simulink model "ASG_algorithm"  (R2024a)
settings: Solver=ode1  StartTime=0.0  StopTime=60  FixedStep=0.01  RelTol=1e-3
libraries: simulink x3
(part 1 of 3)
settings Model: Creator=victo  LastModifiedBy=victo

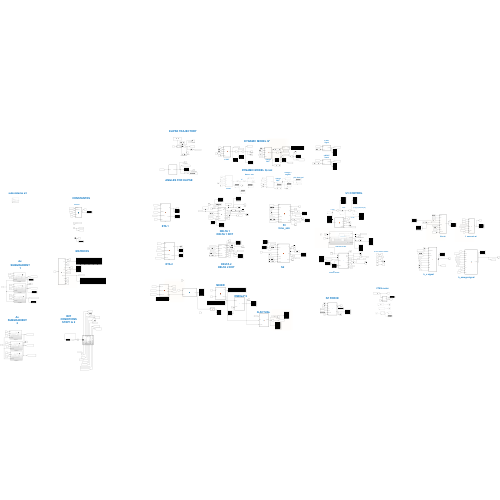
[thumbnail: Simulink's stored preview of the top-level diagram]
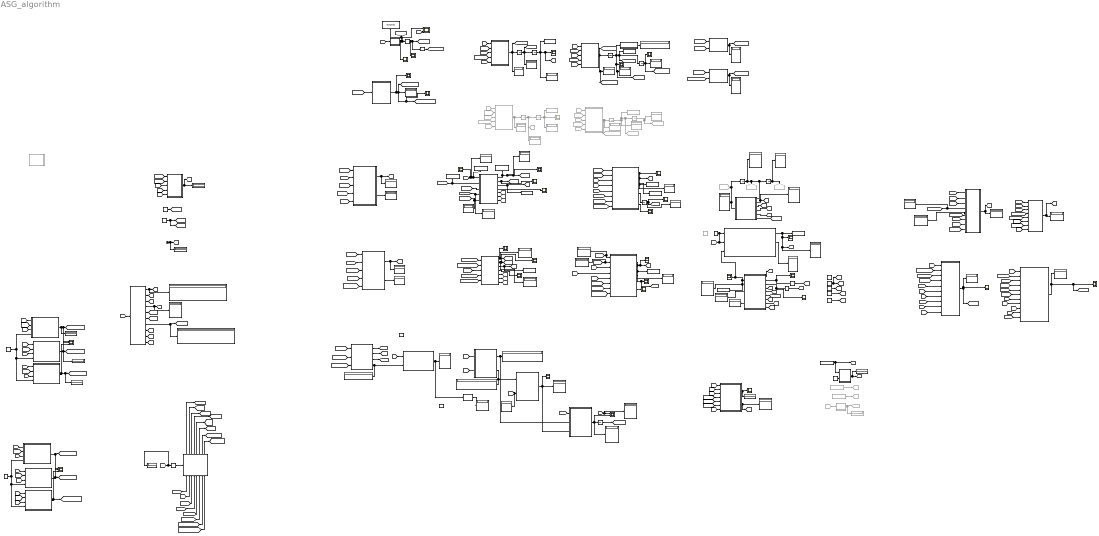
== system ASG_algorithm ==
  note: omega DOT
  note: q_dot
  note: h_omega signal
  note: ETA 2
  note: DYNAMIC MODEL Q*
  note: S1
  note: DELTA 1
      | DELTA 1 DOT
  note: h_v signal
  note: U1 CONTROL
  note: S2
  note: U1
      | CONTROL SIGNAL
  note: MATRICES
  note: Av. SUBGRADIENT 2
  note: S1
      | time_sim
  note: Av. SUBGRADIENT 1
  note: Q = Q*
  note: ELIPSE TRAJECTORY
  note: LOW PASS FILTER
  note: DELTA 2
      | DELTA 2 DOT
  note: fv(v,w)
  note: CONSTANTES
  note: V DOT
  note: f_omega(v,w)
  note: RHO & K1
  note: ETA 1
  note: K1, K2, THETA1, THETA2
  note: ANGLES FOR ELIPSE
  note: INIT CONDITIONS
      | STEP1 & 2
  note: DYNAMIC MODEL Q real
  note: V DOT
  note: omega DOT
  note: S1
  note: Kappa - pos
  note: omega, v angular
  note: phi, theta, psi
  note: q = [x,y,z,phi,theta,psi]
  note: V
  note: q_ddot
  note: MIXER
  note: CTES motor
  note: OMEGA^2
  note: subsistema s3
  note: Q ACTUAL
  note: FZ FORCE
  note: q DOT signal
  note: q DDOT signal
  AverageBlock : Subsystem
  AverageBlock1 : Subsystem
  AverageBlock2 : Subsystem
  AverageBlock3 : Subsystem
  AverageBlock4 : Subsystem
  AverageBlock5 : Subsystem
  Clock : Clock
  Compare To Constant : simulink/Logic and Bit Operations/Compare To Constant  relop===  const=0.0  OutDataTypeStr=boolean
  Constant : Constant  Value=0.5
  Constant1 : Constant  Value=[0;0;0]
  Constant10 : Constant
  Constant14 : Constant  Commented=on  Value=2*10^(-4)
  Constant15 : Constant  Commented=on  Value=1.95*10^(-4)  VectorParams1D=off
  Constant16 : Constant  Value=5  VectorParams1D=off
  Constant2 : Constant  Value=[1;1;1;1]
  Constant3 : Constant  Value=[0;0;6;0;0;0]
  Constant4 : Constant  Value=4  VectorParams1D=off
  Constant5 : Constant  Value=0.03
  Constant7 : Constant  Value=6*10^(-4)
  Constant9 : Constant
  DELTA 1 : Scope
  DELTA 2 : Scope
  DELTA1_DOT : Scope
  DELTA2 DOT4 : Scope
  Derivative1 : Derivative
  Derivative2 : Derivative
  Display{,1..53,64..65,67..69,71,89} (61 alike) : Display
  Display{55,70,73..75,77..78} (7 alike) : Display  Commented=on
  Enabled Subsystem : Subsystem  TreatAsAtomicUnit=on
  From125 : From  Commented=on  GotoTag=FV
  From126 : From  Commented=on  GotoTag=ZERO_I
  From134 : From  Commented=on  GotoTag=I_ZERO
  From146 : From  Commented=on  GotoTag=D_INV
  From147 : From  Commented=on  GotoTag=Q_ACTUAL
  From148 : From  Commented=on  GotoTag=XIsubk
  From157 : From  Commented=on  GotoTag=FW
  From199 : From  Commented=on  GotoTag=JM
  From217 : From  Commented=on  GotoTag=D_INV
  From218 : From  Commented=on  GotoTag=Q_ACTUAL
  From219 : From  Commented=on  GotoTag=XIsubk
  Fz : Scope
  Goto103 : Goto  Commented=on  GotoTag=DM
  Goto104 : Goto  Commented=on  GotoTag=JM
  Goto105 : Goto  Commented=on  GotoTag=JM_INV
  Goto138 : Goto  Commented=on  GotoTag=ANGLES_Q_DOT
  Goto139 : Goto  Commented=on  GotoTag=ANGLES_Q_DDOT
  Goto140 : Goto  Commented=on  GotoTag=V_LIN
  Goto37 : Goto  Commented=on  GotoTag=q_signal
  Goto38 : Goto  Commented=on  GotoTag=q_dot_signal
  Goto47 : Goto  Commented=on  GotoTag=ANGLES_Q
  Goto63 : Goto  Commented=on  GotoTag=q_ddot_signal
  HV : Scope
  HW : Scope
  Integrator{,1..6} (7 alike) : Integrator
  Integrator{9..12} (4 alike) : Integrator  Commented=on
  KAPPA : Scope
  KAPPA POS DESEADA : Scope
  KAPPA REAL1 : Scope
  KAPPA REAL2 : Scope  Commented=on
  KAPPA des : Scope  NumInputPorts=2
  MATLAB Function : MATLAB Function  TreatAsAtomicUnit=on
  MATLAB Function1 : MATLAB Function  TreatAsAtomicUnit=on
  MATLAB Function10 : MATLAB Function  TreatAsAtomicUnit=on
  MATLAB Function11 : MATLAB Function  TreatAsAtomicUnit=on
  MATLAB Function12 : MATLAB Function  TreatAsAtomicUnit=on
  MATLAB Function13 : MATLAB Function  TreatAsAtomicUnit=on
  MATLAB Function14 : MATLAB Function  TreatAsAtomicUnit=on
  MATLAB Function15 : MATLAB Function  TreatAsAtomicUnit=on
  MATLAB Function16 : MATLAB Function  TreatAsAtomicUnit=on
  MATLAB Function17 : MATLAB Function  TreatAsAtomicUnit=on
  MATLAB Function18 : MATLAB Function  TreatAsAtomicUnit=on
  MATLAB Function19 : MATLAB Function  TreatAsAtomicUnit=on
  MATLAB Function2 : MATLAB Function  TreatAsAtomicUnit=on
  MATLAB Function20 : MATLAB Function  TreatAsAtomicUnit=on
  MATLAB Function21 : MATLAB Function  TreatAsAtomicUnit=on
  MATLAB Function22 : MATLAB Function  TreatAsAtomicUnit=on
  MATLAB Function23 : MATLAB Function  TreatAsAtomicUnit=on
  MATLAB Function24 : MATLAB Function  TreatAsAtomicUnit=on
  MATLAB Function25 : MATLAB Function  TreatAsAtomicUnit=on
  MATLAB Function26 : MATLAB Function  Commented=on  TreatAsAtomicUnit=on
  MATLAB Function27 : MATLAB Function  TreatAsAtomicUnit=on
  MATLAB Function28 : MATLAB Function  Commented=on  TreatAsAtomicUnit=on
  MATLAB Function3 : MATLAB Function  TreatAsAtomicUnit=on
  MATLAB Function4 : MATLAB Function  TreatAsAtomicUnit=on
  MATLAB Function45 : MATLAB Function  TreatAsAtomicUnit=on
  MATLAB Function5 : MATLAB Function  Commented=on  TreatAsAtomicUnit=on
  MATLAB Function6 : MATLAB Function  TreatAsAtomicUnit=on
  MATLAB Function7 : MATLAB Function  TreatAsAtomicUnit=on
  MATLAB Function8 : MATLAB Function  TreatAsAtomicUnit=on
  MATLAB Function9 : MATLAB Function  TreatAsAtomicUnit=on
  MIU1 : Constant  Value=0.02
  MIU2 : Constant  Commented=on  Value=0.1
  NORM D1 : Scope
  NORM S1 : Scope
  NORM S2 : Scope
  Norm D2 : Scope
  Q FILTRADA = Q ESTRELLA : Scope
  "Q SIGNAL " : Scope
  Q_comparing : Scope  NumInputPorts=2
  ROTORS VEL : Scope
  S1 : Scope
  S2 : Scope
  SIGN : Signum
  SIGN S1 : Scope
  SIGN S2 : Scope
  Scope1 : Scope  NumInputPorts=3
  Scope2 : Scope  NumInputPorts=3
  Scope3 : Scope
  Scope4 : Scope
  Sign1 : Signum
  Subsystem : Subsystem
  Subsystem1 : Subsystem  Commented=on
  THETA DESIRED : Scope
  THETA DOT DESIRED : Scope
  To Workspace : ToWorkspace  VariableName=dronepos  SampleTime=-1
  To Workspace1 : ToWorkspace  VariableName=simout1  SampleTime=-1
  To Workspace10 : ToWorkspace  VariableName=u1  SaveFormat=Timeseries  SampleTime=-1
  To Workspace11 : ToWorkspace  VariableName=kappad1  SampleTime=-1
  To Workspace13 : ToWorkspace  VariableName=q_star  SampleTime=-1
  To Workspace14 : ToWorkspace  Commented=on  VariableName=droneor1  SampleTime=-1
  To Workspace15 : ToWorkspace  Commented=on  VariableName=dronepos1  SampleTime=-1
  To Workspace2 : ToWorkspace  VariableName=s1  SampleTime=-1
  To Workspace3 : ToWorkspace  VariableName=time_sim  SampleTime=-1
  To Workspace4 : ToWorkspace  VariableName=kappad  SampleTime=-1
  To Workspace5 : ToWorkspace  VariableName=a1  SampleTime=-1
  To Workspace6 : ToWorkspace  VariableName=realkappa  SampleTime=-1
  To Workspace7 : ToWorkspace  VariableName=droneor  SampleTime=-1
  To Workspace8 : ToWorkspace  VariableName=a2  SampleTime=-1
  To Workspace9 : ToWorkspace  VariableName=s2  SampleTime=-1
  Unit Delay : UnitDelay  SampleTime=-1  HasFrameUpgradeWarning=on
  VEL DESEADA : Scope
  ZETA1 : Scope
  ZETA2 : Scope
  eta1 : MATLAB Function  TreatAsAtomicUnit=on
  eta2 : MATLAB Function  TreatAsAtomicUnit=on
  theta1 : Constant  Value=0.01
  theta2 : Constant  Value=0.5
  theta5 : Constant  Value=1e-6
  wires:
  MATLAB Function3/6(a1_y) -> [A1_Y]
  MATLAB Function11/1(fw) -> Display19/1, [FW]
  [TIME] -> MATLAB Function16/10(t)
  [KAPPA] -> Enabled Subsystem/2(kappa)
  [A1] -> MATLAB Function16/6(a1)
  MATLAB Function19/1(s2) -> Display42/1, To Workspace9/1, S2/1, [S2]
  [RHO1] -> MATLAB Function4/5(rho1)
  MATLAB Function6/2(t_s1) -> To Workspace3/1
  Enabled Subsystem/1(v_actual0) -> [V_ACT_0]
  [THETA2] -> MATLAB Function18/6(theta2)
  [V_ACTUAL] -> Display17/1, MATLAB Function10/4(v)
  [THETA2] -> AverageBlock3/2(theta)
  Enabled Subsystem/2(kappa0) -> [KAPPA_0]
  MATLAB Function6/3(Z1) -> Integrator2/1
  Integrator4/1 -> MATLAB Function7/1(vector_rpy), Integrator6/1, To Workspace7/1, [OMEGA_ACTV1], Scope3/1, [ANGLES_Q_DOT], Display21/1
  [THETA_ACTUAL] -> Enabled Subsystem/5(theta_actual)
  [G_Q] -> MATLAB Function10/6(g_q)
  [XIsubk] -> MATLAB Function14/5(xi_subv)
  From217/1 -> MATLAB Function28/3(D_inv)
  MATLAB Function17/1(omega_dot) -> [THETA_ACTUAL_DDOT], [ANGLES_Q_DDOT], Display25/1, Integrator4/1
  MATLAB Function8/6(a2_y) -> [A2_Y]
  MATLAB Function9/6(zero_I) -> [ZERO_I]
  [D_INV] -> MATLAB Function17/3(D_inv)
  From126/1 -> MATLAB Function28/2(zero_I)
  [A2X_AVERAGE] -> MATLAB Function19/6(a2x_average)
  From146/1 -> MATLAB Function5/3(D_inv)
  Integrator11/1 -> To Workspace15/1, KAPPA REAL2/1, Display78/1
  [K1] -> MATLAB Function12/4(k1)
  [THETA2] -> AverageBlock4/2(theta)
  From134/1 -> MATLAB Function5/2(I_zero)
  eta1/2(sum_result) -> Display9/1
  [TIME] -> AverageBlock1/3(t)
  Integrator6/1 -> Scope4/1, [THETA_ACTUAL], Display28/1
  [ETA1] -> MATLAB Function16/7(eta1)
  [S1] -> SIGN/1
  MATLAB Function/1(out) -> Display2/1, Integrator/1, Goto63/1
  AverageBlock5/1(Out1) -> [A2Z_AVERAGE], Scope2/3
  [ZETA1] -> MATLAB Function16/9(zeta1)
  [H_OMEGA] -> MATLAB Function12/6(h_omega)
  [OMEGA_ACTV1] -> MATLAB Function8/4(omega_actual)
  [DELTA1] -> MATLAB Function6/1(delta1)
  [RHO2] -> MATLAB Function12/7(k2)
  eta2/1(eta2) -> [ETA2], Display40/1
  [DELTA1] -> MATLAB Function16/8(delta1)
  [DELTA1_DOT] -> MATLAB Function6/2(delta1_dot)
  [TIME] -> AverageBlock5/3(t)
  [KAPPA] -> KAPPA/1, Display6/1, To Workspace6/1, MATLAB Function3/1(kappa_actual)
  MATLAB Function9/4(g_q) -> Display27/1, [G_Q]
  [A1Z_AVERAGE] -> MATLAB Function6/8(a1z_average)
  From147/1 -> MATLAB Function5/4(Q)
  [D_INV] -> MATLAB Function11/2(D_inv)
  MATLAB Function9/5(I_zero) -> [I_ZERO]
  MATLAB Function5/1(v_dot) -> Integrator9/1, Display73/1
  [S2] -> MATLAB Function12/9(s2)
  [V_ACTUAL] -> MATLAB Function11/4(v)
  [V_DESEADA] -> Display30/1, MATLAB Function3/5(v_desired)
  [TIME] -> MATLAB Function18/7(t)
  MATLAB Function3/5(a1_x) -> [A1_X]
  [C_q] -> MATLAB Function11/3(C)
  MATLAB Function3/2(delta1_dot) -> [DELTA1_DOT], DELTA1_DOT/1
  [S2] -> Sign1/1
  Integrator/1 -> Display4/1, Goto38/1, MATLAB Function/1(q_dot), Integrator1/1
  MATLAB Function8/5(a2_x) -> [A2_X]
  [I_ZERO] -> MATLAB Function14/2(I_zero)
  MATLAB Function8/4(F_d2) -> Norm D2/1
  [THETA2] -> eta2/1(theta2)
  [V_ACTUAL] -> Enabled Subsystem/1(v_actual)
  [A2_Y] -> AverageBlock4/1(In1)
  [FV] -> MATLAB Function16/1(fv)
  AverageBlock/1(Out1) -> Display33/1, [A1X_AVERAGE], Scope1/1
  MATLAB Function16/1(hv) -> [H_V], Display36/1, HV/1
  MATLAB Function3/4(F_d1) -> NORM D1/1
  [KFC0] -> MATLAB Function10/7(kf_c0)
  [KFC0] -> MATLAB Function11/8(Kf_c0)
  [A1_Y] -> AverageBlock1/1(In1)
  Enabled Subsystem/6(thetadot0) -> [THETADOT0]
  [ETA1] -> MATLAB Function6/3(eta1)
  theta2/1 -> [THETA2]
  MATLAB Function12/3(value_s2) -> Display71/1
  [OMEGA_ACTV1] -> MATLAB Function11/5(omega)
  [KAPPA_TRY] -> Enabled Subsystem/4(kappa_try)
  [TIME] -> MATLAB Function20/1(t)
  MATLAB Function21/1(desired_theta) -> THETA DESIRED/1, [DESIRED_THETA_ELIP], THETA DOT DESIRED/1, [DESIRED_DTHETA_ELIP], Display13/1
  Integrator12/1 -> Goto47/1, Display77/1
  Integrator2/1 -> Display/1, ZETA1/1, [ZETA1]
  [Q] -> MATLAB Function14/4(Q)
  [A2_Z] -> AverageBlock5/1(In1)
  [THETA0] -> eta2/2(THETA_0)
  [THETA_ACTUAL] -> MATLAB Function8/1(theta_actual)
  [S1] -> MATLAB Function12/8(s1)
  [THETA1] -> AverageBlock1/2(theta)
  AverageBlock2/1(Out1) -> Display1/1, [A1Z_AVERAGE], Scope1/3
  [TIME] -> MATLAB Function6/4(t)
  Constant1/1 -> [XIsubk], [XIsubk_dot]
  [DELTA2] -> MATLAB Function19/1(delta2), Display7/1
  From125/1 -> MATLAB Function5/1(fv)
  [D_INV] -> MATLAB Function14/3(D_inv)
  eta2/2(sum_result) -> Display41/1
  MATLAB Function12/1(u1) -> To Workspace10/1, Display43/1, "Q SIGNAL "/1, Subsystem/3(U1)
  [D] -> MATLAB Function12/1(D)
  Sign1/1 -> SIGN S2/1, MATLAB Function12/3(sign_s2)
  [DESIRED_DTHETA_ELIP] -> MATLAB Function8/5(omega_desired)
  [FW] -> MATLAB Function18/1(fw)
  [Q] -> MATLAB Function17/4(Q)
  MATLAB Function9/3(C) -> [C_q]
  Constant9/1 -> AverageBlock2/4(constant sign), AverageBlock1/4(constant sign), AverageBlock/4(constant sign)
  [D_INV] -> MATLAB Function10/2(D_inv)
  [A2Y_AVERAGE] -> MATLAB Function19/7(a2y_average)
  [DELTA2_DOT] -> Display65/1, MATLAB Function19/2(delta2_dot)
  Subsystem/1(Q_STAR) -> [Q], Display64/1, Q FILTRADA = Q ESTRELLA/1, To Workspace13/1
  [XIsubk] -> MATLAB Function17/5(xi_subw)
  theta1/1 -> [THETA1]
  Derivative2/1 -> [V_DOT_DESEADA]
  [ZERO_I] -> MATLAB Function17/2(zero_I)
  [EPSILON] -> MATLAB Function8/3(epsilon)
  [A2] -> MATLAB Function18/8(a2)
  [TIME] -> MATLAB Function19/4(t)
  [THETA_DES0] -> eta2/3(THETA_deseada_0)
  [TIME] -> AverageBlock4/3(t)
  AverageBlock4/1(Out1) -> [A2Y_AVERAGE], Scope2/2
  [THETA1] -> MATLAB Function4/4(theta1)
  [TIME] -> Compare To Constant/1, Display51/1
  [THETA1] -> MATLAB Function16/5(theta1)
  Compare To Constant/1 -> Enabled Subsystem/Enable
  [ZETA2] -> MATLAB Function18/5(zeta2)
  [DRAG_MATRIX] -> MATLAB Function/6(drag_matrix)
  [V_ACTUAL] -> MATLAB Function16/3(v_actual)
  [OMEGA_ACTV1] -> MATLAB Function18/2(omega)
  [THETA1] -> eta1/1(theta1)
  [OMEGA_ACTV1] -> Enabled Subsystem/6(omega_actual)
  [THETA1] -> MATLAB Function6/5(theta1)
  MATLAB Function7/1(R_graph) -> Display26/1
  [KAPPA_TRY] -> To Workspace4/1, MATLAB Function3/2(kappa_desired)
  [C_q] -> MATLAB Function/4(C_q)
  MIU1/1 -> [MIU], Subsystem/2(MIU2), Subsystem/1(MIU1)
  [THETADOT_DES0] -> eta2/5(THETA_DOT_0)
  theta5/1 -> [EPSILON]
  [DELTA2] -> MATLAB Function18/3(delta2)
  [TIME] -> AverageBlock2/3(t)
  [A1_Z] -> AverageBlock2/1(a1_z)
  [DRAG_MATRIX] -> MATLAB Function11/7(drag_matrix)
  [V_ACT_0] -> eta1/2(v_0)
  AverageBlock1/1(Out1) -> Scope1/2, Display29/1, [A1Y_AVERAGE]
  [KAPPA] -> KAPPA des/2
  [FW] -> MATLAB Function17/1(fw)
  Integrator10/1 -> To Workspace14/1, Goto138/1, Integrator12/1, Display74/1
  MATLAB Function19/2(Z2) -> [ZETA2], ZETA2/1
  MATLAB Function20/1(kappa) -> KAPPA des/1, Derivative1/1, To Workspace11/1, [KAPPA_TRY], KAPPA POS DESEADA/1
  Enabled Subsystem/8(thetadot_desired0) -> [THETADOT_DES0]
  MATLAB Function10/1(fv) -> [FV], Display23/1
  [OMEGA_ACTV1] -> Display18/1, MATLAB Function10/5(omega)
  MATLAB Function6/4(norm_s1) -> NORM S1/1
  Integrator1/1 -> Display3/1, Goto37/1
  SIGN/1 -> MATLAB Function12/2(sign_s1), SIGN S1/1
  [ZERO_I] -> MATLAB Function18/11(zero_I)
  [THETA2] -> MATLAB Function19/5(theta2)
  [TIME] -> MATLAB Function4/3(t)
  [A2Z_AVERAGE] -> MATLAB Function19/8(a2z_average)
  MATLAB Function9/8(l_arm) -> [L_ARM]
  [THETADOT0] -> eta2/4(THETA_DOT_desired_0)
  MATLAB Function9/7(drag_matrix) -> Display53/1, [DRAG_MATRIX]
  [D_INV] -> MATLAB Function18/9(D_inv)
  [XIsubk] -> MATLAB Function4/1(xi_subkappa)
  [A2_X] -> AverageBlock3/1(a2_x)
  MATLAB Function12/2(value_s1) -> Display68/1
  [DESIRED_THETA_ELIP] -> Enabled Subsystem/7(theta_desired)
  [KAPPA_0] -> eta1/5(kappa_0)
  Derivative1/1 -> VEL DESEADA/1, [V_DESEADA], Derivative2/1
  [TIME] -> AverageBlock3/3(t)
  [KA] -> MATLAB Function9/1("Ka ")
  [THETA1] -> AverageBlock2/2(theta)
  eta1/1(eta1) -> [ETA1], Display5/1
  [DESIRED_DTHETA_ELIP] -> Enabled Subsystem/8(thetadot_desired)
  [KAPPAD0] -> eta1/4(kappa_desired_0)
  [G_Q] -> MATLAB Function11/6(g_q)
  [XIsubk_dot] -> MATLAB Function4/2(xi_subkappa_dot)
  [TIME] -> AverageBlock/3(t)
  [V_DESEADA] -> MATLAB Function16/4(v_deseada)
  MATLAB Function8/2(delta2_dot) -> Display39/1, DELTA2 DOT4/1, [DELTA2_DOT]
  MATLAB Function9/1(D) -> Display24/1, [D]
  [A1_X] -> AverageBlock/1(a1_x)
  [EPSILON] -> MATLAB Function3/3(epsilon)
  [A1X_AVERAGE] -> MATLAB Function6/6(a1x_average)
  [C_q] -> MATLAB Function10/3(C)
  Enabled Subsystem/3(vdesired0) -> [V_DESIRED0]
  [G_Q] -> MATLAB Function/5(g_q)
  Constant10/1 -> AverageBlock3/4(constant sign), AverageBlock5/4(constant sign), AverageBlock4/4(constant sign)
  MATLAB Function6/1(s1) -> Display10/1, To Workspace2/1, [S1], S1/1
  [A1Y_AVERAGE] -> MATLAB Function6/7(a1y_average)
  [DESIRED_THETA_ELIP] -> MATLAB Function8/2(theta_desired)
  From219/1 -> MATLAB Function28/5(xi_subw)
  Integrator5/1 -> [KAPPA], KAPPA REAL1/1, Display31/1, To Workspace/1
  [H_V] -> MATLAB Function12/5(h_v)
  [Q] -> MATLAB Function18/10(Q)
  MATLAB Function14/1(v_dot) -> [V_DOT_ACTUAL], Display20/1, Integrator3/1
  Enabled Subsystem/5(theta0) -> [THETA0]
  Enabled Subsystem/7(theta_desired0) -> [THETA_DES0]
  [V_DESIRED0] -> eta1/3(v_deseada_0)
  [I_ZERO] -> MATLAB Function10/1(I_zero)
  MATLAB Function3/7(a1_z) -> [A1_Z]
  [ZERO_I] -> MATLAB Function11/1(zero_I)
  [V_ACTUAL] -> Display14/1, MATLAB Function3/4(v_actual)
  From148/1 -> MATLAB Function5/5(xi_subv)
  Enabled Subsystem/4(kappaD0) -> [KAPPAD0]
  [V_DESEADA] -> MATLAB Function21/1(des_vel)
  [V_DOT_DESEADA] -> MATLAB Function16/2(v_dot_deseada)
  [D_INV] -> MATLAB Function/3(D_inv)
  Constant/1 -> [KA]
  From218/1 -> MATLAB Function28/4(Q)
  [THETA2] -> AverageBlock5/2(theta)
  [FV] -> MATLAB Function14/1(fv)
  From157/1 -> MATLAB Function28/1(fw)
  Integrator9/1 -> Goto140/1, Integrator11/1, Display70/1
  Integrator3/1 -> Integrator5/1, Display16/1, [V_ACTUAL]
  MATLAB Function3/3(a1) -> [A1], To Workspace5/1
  [THETA1] -> AverageBlock/2(theta)
  [V_DESEADA] -> Enabled Subsystem/3(v_desired)
  AverageBlock3/1(Out1) -> [A2X_AVERAGE], Scope2/1
  MATLAB Function3/1(delta1) -> DELTA 1/1, Display11/1, [DELTA1], To Workspace1/1
  MATLAB Function8/3(a2) -> To Workspace8/1, [A2]
  [DRAG_MATRIX] -> MATLAB Function10/8(drag_matrix)
  MATLAB Function19/3(norm_s2) -> NORM S2/1
  MATLAB Function9/2(D_inv) -> [D_INV]
  Constant4/1 -> [RHO1], [RHO2]
  Subsystem/2(Q_DOT_STAR) -> Display69/1
  [ETA2] -> MATLAB Function19/3(eta2)
  MATLAB Function18/1(h_omega) -> [H_OMEGA], HW/1, Display35/1
  MATLAB Function28/1(omega_dot) -> Integrator10/1, Display75/1, Goto139/1
  MATLAB Function4/1(k1) -> Display12/1, [K1]
  [ETA2] -> MATLAB Function18/4(eta2)
  MATLAB Function8/7(a2_z) -> [A2_Z]
  Clock/1 -> Display52/1, [TIME]
  MATLAB Function8/1(delta2) -> DELTA 2/1, Display38/1, [DELTA2]
  [Q] -> MATLAB Function/2(Q), Display67/1
  [V_ACTUAL] -> MATLAB Function45/1(v_lin)
  [OMEGA_ACTV1] -> MATLAB Function45/2(v_ang)
  MATLAB Function45/1(q_dot_signal) -> Display89/1, [q_dot_signal]
  [KV] -> MATLAB Function1/1(Kv)
  [KM] -> MATLAB Function1/2(Km)
  Constant14/1 -> Goto103/1
  From199/1 -> MATLAB Function26/1(Jm)
  Constant15/1 -> Goto104/1
  Constant7/1 -> MATLAB Function27/1(Kv), [KV]
  MATLAB Function26/1(Jm_inv) -> Goto105/1, Display55/1
  MATLAB Function1/1(mixer) -> MATLAB Function23/2(mixer), Display8/1
  MATLAB Function1/2(mixer_inv) -> MATLAB Function2/1(mixer_inv), Display15/1
  [THETA_ACTUAL] -> MATLAB Function15/1(angles_vector)
  MATLAB Function15/2(R_dot) -> [R3_DOT]
  MATLAB Function15/1(R) -> [R3]
  MATLAB Function15/3(R_ddot) -> [R3_DDOT]
  [ANGLES_Q_DOT] -> MATLAB Function15/2(anglesdot_vector)
  [ANGLES_Q_DDOT] -> MATLAB Function15/3(anglesddot_vector)
  MATLAB Function15/4(R_inv) -> MATLAB Function13/2(R_inv), Display22/1
  MATLAB Function13/1(Q_6X1) -> MATLAB Function22/1(Q6x1), Display32/1
  MATLAB Function22/1(Q4x1) -> Display47/1
  MATLAB Function2/1(rotors_vel) -> MATLAB Function23/3(rotors_vel4x1), ROTORS VEL/1, Display34/1
  [R3] -> MATLAB Function23/1(R)
  MATLAB Function23/1(Q_actual) -> Unit Delay/1, Q_comparing/2, Display37/1
  [Q] -> Q_comparing/1, Display48/1
  [Q] -> MATLAB Function13/1(Q)
  Unit Delay/1 -> [Q_actual]
  MATLAB Function9/9(M) -> [Masa]
  MATLAB Function9/10(g) -> [G_cte]
  [V_DOT_ACTUAL] -> MATLAB Function25/1(v_lin)
  MATLAB Function25/1(q_dot_signal) -> Display44/1, [q_ddot_signal]
  [ANGLES_Q_DDOT] -> MATLAB Function25/2(v_ang)
  [Masa] -> MATLAB Function24/1(M)
  [G_cte] -> MATLAB Function24/2(g)
  [KA] -> MATLAB Function24/3(Ka)
  [q_dot_signal] -> MATLAB Function24/4(q_dot)
  [q_ddot_signal] -> MATLAB Function24/5(q_ddot)
  [THETA_ACTUAL] -> MATLAB Function24/6(theta_actual)
  MATLAB Function24/1(Fz) -> Display45/1, Fz/1
  [Q] -> MATLAB Function24/7(Q6)
  MATLAB Function24/2(Q4) -> [Q4], Display46/1
  [Q4] -> Display49/1, MATLAB Function2/2(control4x1)
  MATLAB Function27/1(Km) -> Display50/1, [KM]
  Constant5/1 -> MATLAB Function27/2(porcent_force)

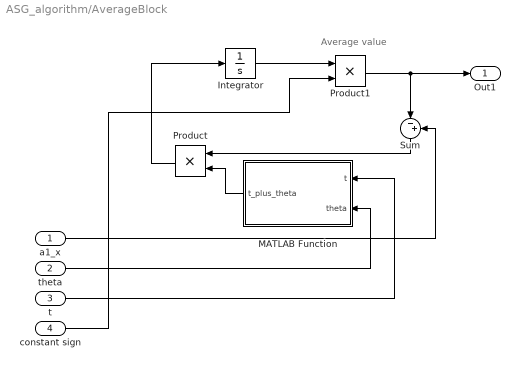
== system ASG_algorithm/AverageBlock ==
  note: Average value
  a1_x : Inport
  theta : Inport  Port=2
  t : Inport  Port=3
  constant sign : Inport  Port=4
  Integrator : Integrator
  MATLAB Function : MATLAB Function  TreatAsAtomicUnit=on
  Product : Product
  Product1 : Product
  Sum : Sum  Inputs=|-+
  Out1 : Outport
  wires:
  MATLAB Function/1(t_plus_theta) -> Product/2
  Sum/1 -> Product/1
  Product/1 -> Integrator/1
  theta/1 -> MATLAB Function/2(theta)
  a1_x/1 -> Sum/2
  t/1 -> MATLAB Function/1(t)
  Integrator/1 -> Product1/1
  Product1/1 -> Out1/1, Sum/1
  constant sign/1 -> Product1/2

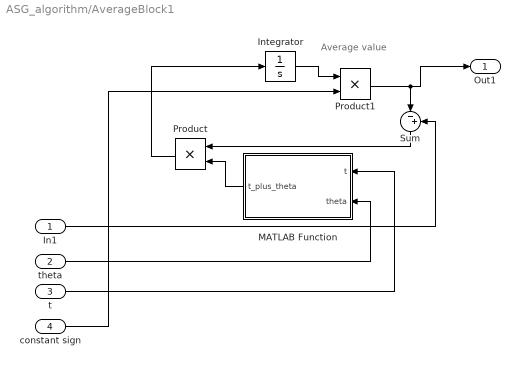
== system ASG_algorithm/AverageBlock1 ==
  note: Average value
  In1 : Inport
  theta : Inport  Port=2
  t : Inport  Port=3
  constant sign : Inport  Port=4
  Integrator : Integrator
  MATLAB Function : MATLAB Function  TreatAsAtomicUnit=on
  Product : Product
  Product1 : Product
  Sum : Sum  Inputs=|-+
  Out1 : Outport
  wires:
  MATLAB Function/1(t_plus_theta) -> Product/2
  Sum/1 -> Product/1
  Product/1 -> Integrator/1
  theta/1 -> MATLAB Function/2(theta)
  In1/1 -> Sum/2
  t/1 -> MATLAB Function/1(t)
  Product1/1 -> Sum/1, Out1/1
  Integrator/1 -> Product1/1
  constant sign/1 -> Product1/2

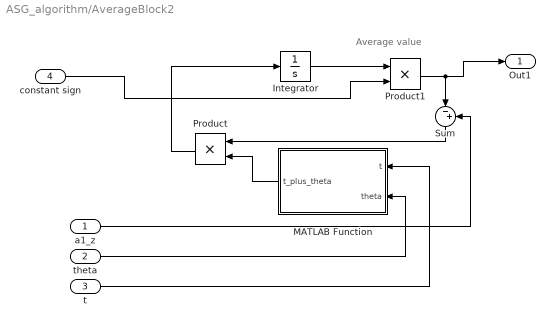
== system ASG_algorithm/AverageBlock2 ==
  note: Average value
  a1_z : Inport
  theta : Inport  Port=2
  t : Inport  Port=3
  constant sign : Inport  Port=4
  Integrator : Integrator
  MATLAB Function : MATLAB Function  TreatAsAtomicUnit=on
  Product : Product
  Product1 : Product
  Sum : Sum  Inputs=|-+
  Out1 : Outport
  wires:
  MATLAB Function/1(t_plus_theta) -> Product/2
  Sum/1 -> Product/1
  Product/1 -> Integrator/1
  theta/1 -> MATLAB Function/2(theta)
  a1_z/1 -> Sum/2
  t/1 -> MATLAB Function/1(t)
  Integrator/1 -> Product1/1
  Product1/1 -> Sum/1, Out1/1
  constant sign/1 -> Product1/2

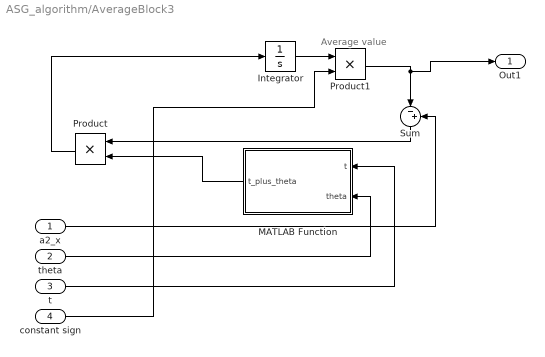
== system ASG_algorithm/AverageBlock3 ==
  note: Average value
  a2_x : Inport
  theta : Inport  Port=2
  t : Inport  Port=3
  constant sign : Inport  Port=4
  Integrator : Integrator
  MATLAB Function : MATLAB Function  TreatAsAtomicUnit=on
  Product : Product
  Product1 : Product
  Sum : Sum  Inputs=|-+
  Out1 : Outport
  wires:
  MATLAB Function/1(t_plus_theta) -> Product/2
  Sum/1 -> Product/1
  Product/1 -> Integrator/1
  theta/1 -> MATLAB Function/2(theta)
  a2_x/1 -> Sum/2
  t/1 -> MATLAB Function/1(t)
  Integrator/1 -> Product1/1
  constant sign/1 -> Product1/2
  Product1/1 -> Sum/1, Out1/1

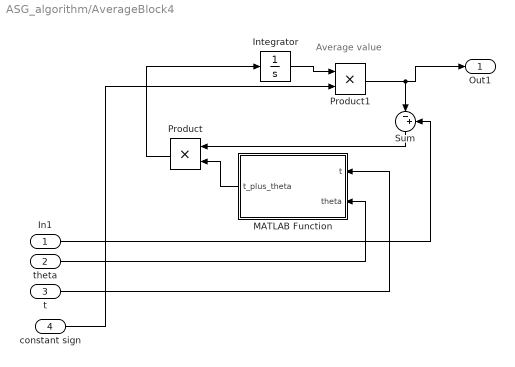
== system ASG_algorithm/AverageBlock4 ==
  note: Average value
  In1 : Inport
  theta : Inport  Port=2
  t : Inport  Port=3
  constant sign : Inport  Port=4
  Integrator : Integrator
  MATLAB Function : MATLAB Function  TreatAsAtomicUnit=on
  Product : Product
  Product1 : Product
  Sum : Sum  Inputs=|-+
  Out1 : Outport
  wires:
  MATLAB Function/1(t_plus_theta) -> Product/2
  Sum/1 -> Product/1
  Product/1 -> Integrator/1
  theta/1 -> MATLAB Function/2(theta)
  In1/1 -> Sum/2
  t/1 -> MATLAB Function/1(t)
  Integrator/1 -> Product1/1
  Product1/1 -> Sum/1, Out1/1
  constant sign/1 -> Product1/2

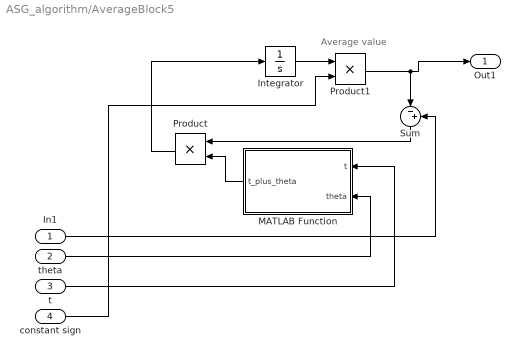
== system ASG_algorithm/AverageBlock5 ==
  note: Average value
  In1 : Inport
  theta : Inport  Port=2
  t : Inport  Port=3
  constant sign : Inport  Port=4
  Integrator : Integrator
  MATLAB Function : MATLAB Function  TreatAsAtomicUnit=on
  Product : Product
  Product1 : Product
  Sum : Sum  Inputs=|-+
  Out1 : Outport
  wires:
  MATLAB Function/1(t_plus_theta) -> Product/2
  Sum/1 -> Product/1
  Product/1 -> Integrator/1
  theta/1 -> MATLAB Function/2(theta)
  In1/1 -> Sum/2
  t/1 -> MATLAB Function/1(t)
  Integrator/1 -> Product1/1
  Product1/1 -> Sum/1, Out1/1
  constant sign/1 -> Product1/2

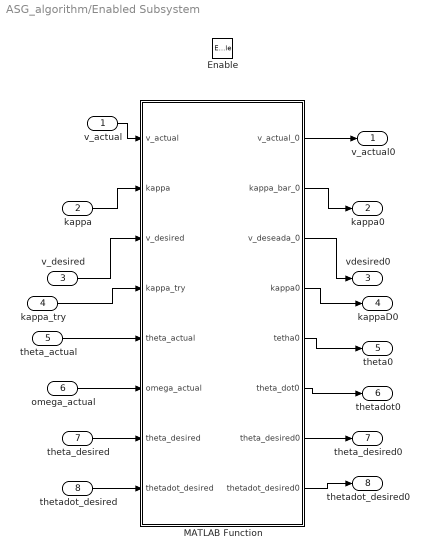
== system ASG_algorithm/Enabled Subsystem ==
  v_actual : Inport
  kappa : Inport  Port=2
  v_desired : Inport  Port=3
  kappa_try : Inport  Port=4
  theta_actual : Inport  Port=5
  omega_actual : Inport  Port=6
  theta_desired : Inport  Port=7
  thetadot_desired : Inport  Port=8
  Enable : EnablePort
  MATLAB Function : MATLAB Function  TreatAsAtomicUnit=on
  v_actual0 : Outport
  kappa0 : Outport  Port=2
  vdesired0 : Outport  Port=3
  kappaD0 : Outport  Port=4
  theta0 : Outport  Port=5
  thetadot0 : Outport  Port=6
  theta_desired0 : Outport  Port=7
  thetadot_desired0 : Outport  Port=8
  wires:
  v_actual/1 -> MATLAB Function/1(v_actual)
  kappa/1 -> MATLAB Function/2(kappa)
  MATLAB Function/2(kappa_bar_0) -> kappa0/1
  MATLAB Function/1(v_actual_0) -> v_actual0/1
  v_desired/1 -> MATLAB Function/3(v_desired)
  MATLAB Function/3(v_deseada_0) -> vdesired0/1
  kappa_try/1 -> MATLAB Function/4(kappa_try)
  MATLAB Function/4(kappa0) -> kappaD0/1
  MATLAB Function/5(tetha0) -> theta0/1
  MATLAB Function/6(theta_dot0) -> thetadot0/1
  theta_actual/1 -> MATLAB Function/5(theta_actual)
  omega_actual/1 -> MATLAB Function/6(omega_actual)
  theta_desired/1 -> MATLAB Function/7(theta_desired)
  thetadot_desired/1 -> MATLAB Function/8(thetadot_desired)
  MATLAB Function/7(theta_desired0) -> theta_desired0/1
  MATLAB Function/8(thetadot_desired0) -> thetadot_desired0/1

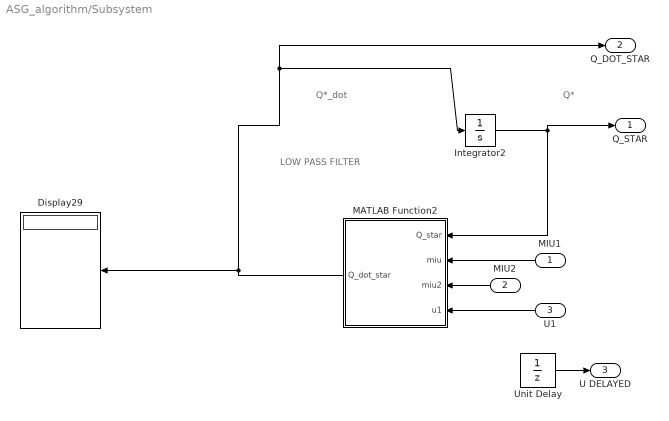
== system ASG_algorithm/Subsystem ==
  note: LOW PASS FILTER
  note: Q*_dot
  note: Q*
  MIU1 : Inport
  MIU2 : Inport  Port=2
  U1 : Inport  Port=3
  Display29 : Display
  Integrator2 : Integrator  UpperSaturationLimit=10  LowerSaturationLimit=-10  IgnoreLimit=on
  MATLAB Function2 : MATLAB Function  TreatAsAtomicUnit=on
  Unit Delay : UnitDelay  SampleTime=-1  HasFrameUpgradeWarning=on
  Q_STAR : Outport
  Q_DOT_STAR : Outport  Port=2
  U DELAYED : Outport  Port=3
  wires:
  MATLAB Function2/1(Q_dot_star) -> Q_DOT_STAR/1, Integrator2/1, Display29/1
  MIU1/1 -> MATLAB Function2/2(miu)
  U1/1 -> MATLAB Function2/4(u1)
  Integrator2/1 -> Q_STAR/1, MATLAB Function2/1(Q_star)
  MIU2/1 -> MATLAB Function2/3(miu2)
  Unit Delay/1 -> U DELAYED/1
